simulink model "SecRwRtStOccupyChk"  (R2018b)
settings: Solver=FixedStepDiscrete  StartTime=0.0  StopTime=10.0  FixedStep=0.01  RelTol=1e-3
undefined symbols (not defined in the file or in its folder): SeatOccupiedSts1
settings Model: Creator=sn2xws  LastModifiedBy=sn2xws
settings DataIOCC: SaveFormat=StructureWithTime
settings OptimizationCC: DefaultParameterBehavior=Inlined  EnhancedBackFolding=on  PassReuseOutputArgsAs=Individual arguments  ZeroExternalMemoryAtStartup=off  ZeroInternalMemoryAtStartup=off  OptimizeBlockOrder=speed  DifferentSizesBufferReuse=on  OptimizationCustomize=off
settings DebuggingCC: ParameterTunabilityLossMsg=error
settings ModelReferenceCC: ModelReferenceNumInstancesAllowed=Single
settings SFSimCC: MATLABDynamicMemAlloc=off
settings RTWCC: SystemTargetFile=autosar.tlc  GenCodeOnly=on  TemplateMakefile=ert_default_tmf  Description=AUTOSAR  GenerateReport=on  IncludeHyperlinkInReport=on  LaunchReport=on  GenerateTraceInfo=on  GenerateTraceReport=on  GenerateTraceReportSl=on  GenerateTraceReportSf=on  GenerateTraceReportEml=on
settings CodeAppCC: ForceParamTrailComments=on  IgnoreCustomStorageClasses=off  OperatorAnnotations=on  SimulinkDataObjDesc=on  SFDataObjDesc=on  InsertBlockDesc=on
settings STFCustomTargetCC: TargetLangStandard=C99 (ISO)  MultiwordLength=256  ParMdlRefBuildCompliant=on  CompOptLevelCompliant=on  IncludeMdlTerminateFcn=off  CombineOutputUpdateFcns=on  SuppressErrorStatus=on  ERTCustomFileBanners=on  SupportNonFinite=off  SupportComplex=off  SupportContinuousTime=off  SupportNonInlinedSFcns=off  RemoveResetFunc=on  MATLABClassNameForMDSCustomization=Simulink.SoftwareTarget.ERTCustomization  AutosarCompliant=on  UseToolchainInfoCompliant=on  LookupTableObjectStructAxisOrder=2,1,3,4,...  LUTObjectStructOrderEvenSpacing=Size,Table,Breakpoints  SystemTargetFile=autosar.tlc
settings ERTTargetCC: TargetLangStandard=C99 (ISO)  ConcurrentExecutionCompliant=off  IncludeMdlTerminateFcn=off  SuppressErrorStatus=on  SupportNonFinite=off  SupportComplex=off  ModelStepFunctionPrototypeControlCompliant=off  CPPClassGenCompliant=off  AutosarCompliant=on  LookupTableObjectStructAxisOrder=2,1,3,4,...  LUTObjectStructOrderEvenSpacing=Size,Table,Breakpoints  InlinedParameterPlacement=NonHierarchical  ERTCustomFileTemplate=example_file_process.tlc  ERTFilePackagingFormat=Compact

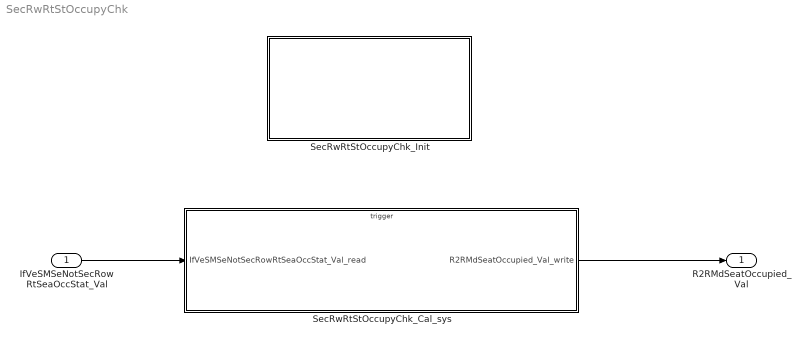
== system SecRwRtStOccupyChk ==
  IfVeSMSeNotSecRowRtSeaOccStat_Val : Inport  OutDataTypeStr=Enum: SeatOccupiedSts1  PortDimensions=1
  SecRwRtStOccupyChk_Cal_sys : Subsystem
  SecRwRtStOccupyChk_Init : Subsystem
  R2RMdSeatOccupied_Val : Outport  OutDataTypeStr=boolean  PortDimensions=1
  wires:
  IfVeSMSeNotSecRowRtSeaOccStat_Val/1 -> SecRwRtStOccupyChk_Cal_sys/1(IfVeSMSeNotSecRowRtSeaOccStat_Val_read)
  SecRwRtStOccupyChk_Cal_sys/1(R2RMdSeatOccupied_Val_write) -> R2RMdSeatOccupied_Val/1

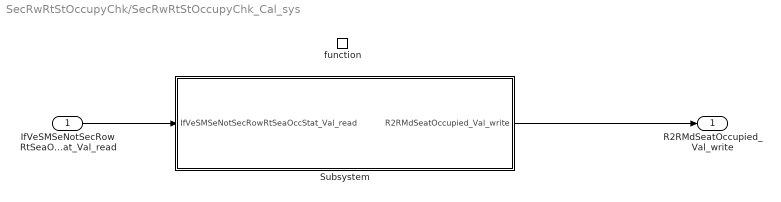
== system SecRwRtStOccupyChk/SecRwRtStOccupyChk_Cal_sys ==
  IfVeSMSeNotSecRowRtSeaOccStat_Val_read : Inport
  function : TriggerPort  TriggerType=function-call  IsSimulinkFunction=on  FunctionName=SecRwRtStOccupyChk_Cal  VariantControl=(inherit)
  Subsystem : Subsystem
  R2RMdSeatOccupied_Val_write : Outport
      settings: EnsureOutportIsVirtual=on
  wires:
  IfVeSMSeNotSecRowRtSeaOccStat_Val_read/1 -> Subsystem/1(IfVeSMSeNotSecRowRtSeaOccStat_Val_read)
  Subsystem/1(R2RMdSeatOccupied_Val_write) -> R2RMdSeatOccupied_Val_write/1

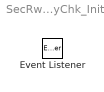
== system SecRwRtStOccupyChk/SecRwRtStOccupyChk_Init ==
  Event Listener : EventListener  EventName=reset

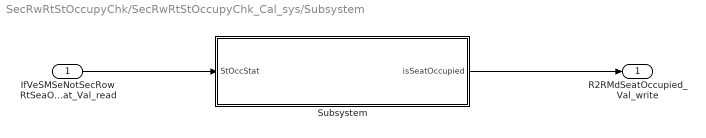
== system SecRwRtStOccupyChk/SecRwRtStOccupyChk_Cal_sys/Subsystem ==
  IfVeSMSeNotSecRowRtSeaOccStat_Val_read : Inport
  Subsystem : Subsystem
  R2RMdSeatOccupied_Val_write : Outport
      settings: EnsureOutportIsVirtual=on
  wires:
  Subsystem/1(isSeatOccupied) -> R2RMdSeatOccupied_Val_write/1
  IfVeSMSeNotSecRowRtSeaOccStat_Val_read/1 -> Subsystem/1(StOccStat)

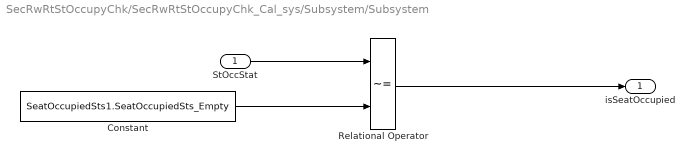
== system SecRwRtStOccupyChk/SecRwRtStOccupyChk_Cal_sys/Subsystem/Subsystem ==
  StOccStat : Inport
  Constant : Constant  Value=SeatOccupiedSts1.SeatOccupiedSts_Empty  OutDataTypeStr=Enum:SeatOccupiedSts1
  Relational Operator : RelationalOperator  Operator=~=  OutDataTypeStr=boolean  RndMeth=Simplest
  isSeatOccupied : Outport  VectorParamsAs1DForOutWhenUnconnected=on
  wires:
  Constant/1 -> Relational Operator/2
  StOccStat/1 -> Relational Operator/1
  Relational Operator/1 -> isSeatOccupied/1
